simulink model "Simulink_DBL"  (R2021b)
settings: Solver=VariableStepAuto  StartTime=0.0  StopTime=10.0  RelTol=1e-3
settings Model: Creator=enrique  LastModifiedBy=enrique
settings SolverCC: AlgebraicLoopSolver=TrustRegion
settings DebuggingCC: SFMachineParentedDataDiag=warning

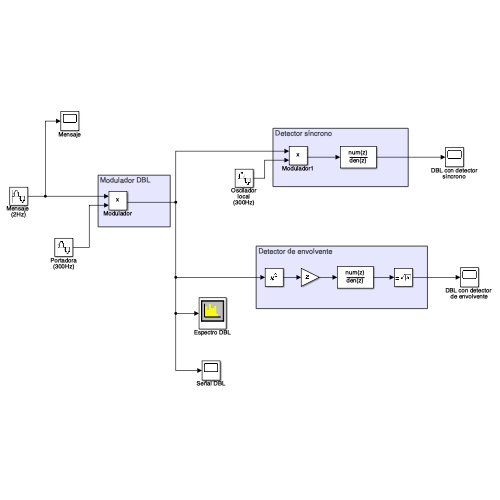
[thumbnail: Simulink's stored preview of the top-level diagram]
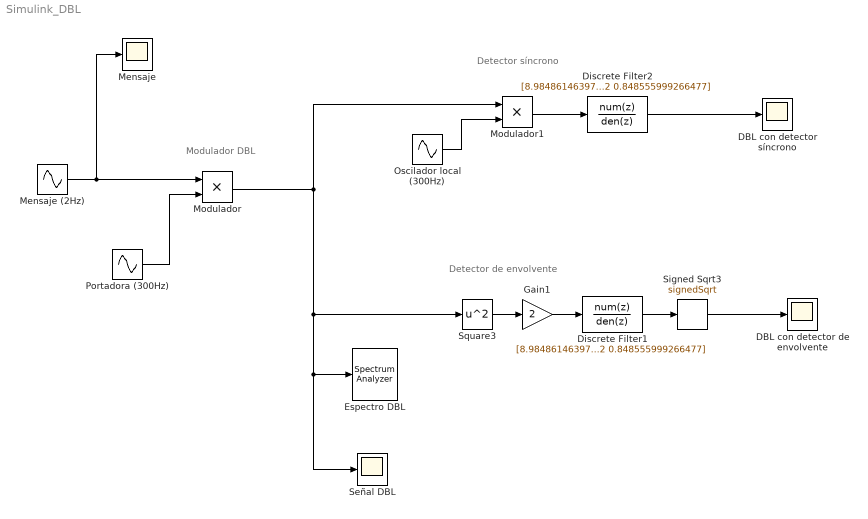
== system Simulink_DBL ==
  note: Detector de envolvente
  note: Detector síncrono
  note: Modulador DBL
  DBL con detector síncrono : Scope
  DBL con detector de envolvente : Scope
  Discrete Filter1 : DiscreteFilter  Numerator="[8.98486146397045e-07\t3.59394458558818e-06\t5.39091687838227e-06\t3.59394458558818e-06\t8.98486146397045e-07]"  Denominator="[1\t-3.83582554064735\t5.52081913662223\t-3.53353521946302\t0.848555999266477]"  InputProcessing=Columns as channels (frame based)
  Discrete Filter2 : DiscreteFilter  Numerator="[8.98486146397045e-07\t3.59394458558818e-06\t5.39091687838227e-06\t3.59394458558818e-06\t8.98486146397045e-07]"  Denominator="[1\t-3.83582554064735\t5.52081913662223\t-3.53353521946302\t0.848555999266477]"  InputProcessing=Columns as channels (frame based)
  Espectro DBL : SpectrumAnalyzer
  Gain1 : Gain  Gain=2
  Mensaje : Scope
  "Mensaje (2Hz) " : Sin  Frequency=2*pi*2  SampleTime=1/5000
  Modulador : Product  OutDataTypeStr=Inherit: Same as first input
  Modulador1 : Product  OutDataTypeStr=Inherit: Same as first input
  Oscilador local (300Hz) : Sin  Amplitude=2  Frequency=2*pi*300  SampleTime=1/5000
  "Portadora (300Hz) " : Sin  Frequency=2*pi*300  SampleTime=1/5000
  Señal DBL : Scope
  Signed Sqrt3 : Sqrt  Operator=signedSqrt  SaturateOnIntegerOverflow=on
  Square3 : Math  Operator=square  SaturateOnIntegerOverflow=on
  wires:
  Discrete Filter2/1 -> DBL con detector síncrono/1
  Signed Sqrt3/1 -> DBL con detector de envolvente/1
  "Mensaje (2Hz) "/1 -> Mensaje/1, Modulador/1
  "Portadora (300Hz) "/1 -> Modulador/2
  Oscilador local (300Hz)/1 -> Modulador1/2
  Modulador1/1 -> Discrete Filter2/1
  Discrete Filter1/1 -> Signed Sqrt3/1
  Square3/1 -> Gain1/1
  Gain1/1 -> Discrete Filter1/1
  Modulador/1 -> Espectro DBL/1, Señal DBL/1, Square3/1, Modulador1/1
